simulink model "trail2_SIGNAL_B"  (R2020b)
settings: Solver=FixedStepAuto  StartTime=0.0  StopTime=60  FixedStep=10  RelTol=1e-3
undefined symbols (not defined in the file or in its folder): sigbuilder_block
libraries: simulink x2
settings Model: Creator=99003785  LastModifiedBy=99003785

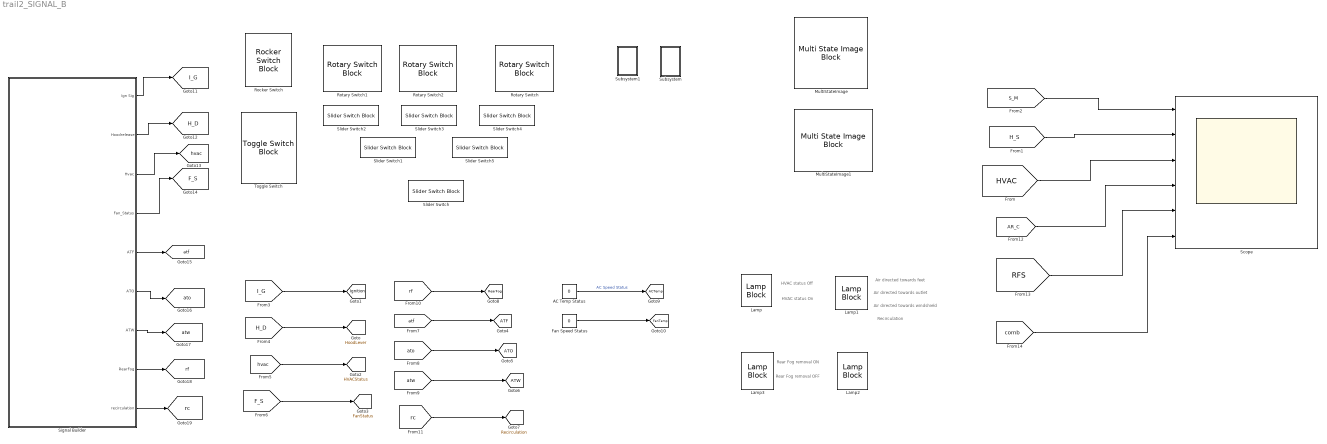
== system trail2_SIGNAL_B ==
  note: Rear Fog removal OFF
  note: Recirculation
  note: Air directed towards feet
  note: Air directed towards outlet
  note: Air directed towards windshield
  note: HVAC status On
  note: Rear Fog removal ON
  note: HVAC status Off
  AC Temp Status : Constant  Value=0
  Fan Speed Status : Constant  Value=0
  Lamp{,1..3} (4 alike) : LampBlock
  MultiStateImage : MultiStateImageBlock
  MultiStateImage1 : MultiStateImageBlock
  Rocker Switch : RockerSwitchBlock
      settings: Values={{'On', 'Off'}, [1 0]}
  Rotary Switch : RotarySwitchBlock
      settings: Values={{'Off', 'Low', 'Medium', 'High'}, [0 1 2 3]}
  Rotary Switch1 : RotarySwitchBlock
      settings: Values={{'Off', 'Low', 'Medium', 'High'}, [0 1 2 3]}
  Rotary Switch2 : RotarySwitchBlock
      settings: Values={{'Off', 'AC', 'Heater', 'Air-Vent'}, [0 1 2 3]}
  Scope : Scope  NumInputPorts=6
  Signal Builder : Subsystem  Tag=STV Subsys  LoadFcn=sigbuilder_block('load');  StartFcn=sigbuilder_block('start');  StopFcn=sigbuilder_block('stop');  ClipboardFcn=sigbuilder_block('clipboard');  mask(Sigbuilder block){tuvar=[0:10]}
      mask help: Simulink:masks:SigbuilderBlock_MD
      mask init:
      | if ~strcmp(get_param(bdroot(gcbh),'SimulationStatus'),'stopped') tuvar = sigbuilder_block('maskInit'); end
      settings: CopyFcn=sigbuilder_block('copy');  DeleteFcn=sigbuilder_block('delete');  ModelCloseFcn=sigbuilder_block('modelClose');  PreSaveFcn=sigbuilder_block('preSave');  PauseFcn=sigbuilder_block('pause');  ContinueFcn=sigbuilder_block('continue');  NameChangeFcn=sigbuilder_block('namechange');  OpenFcn=sigbuilder_block('open',[11.25 5.25 1428 681.75 ]);  CloseFcn=sigbuilder_block('close');
      mask Display: plot(0, 0, 100, 100,[2, 2, 32, 32, 2], [68, 8, 8, 68, 68],[32, 2], [38, 38], [32, 19, 2],[53, 60, 44], [32, 17, 17, 2],[16, 16, 31, 31]);txt = getActiveGroup(gcbh);text(2, 100, txt,'verticalAlignment', 'top');
  Slider Switch{,1..5} (6 alike) : SliderSwitchBlock
      settings: Values={{'Off', 'On'}, [0 1]}
  Subsystem : Subsystem
  Subsystem1 : Subsystem
  Toggle Switch : ToggleSwitchBlock
      settings: Values={{'Off', 'On'}, [0 1]}
  tag scope: ACTemp=global, ATF=global, ATO=global, ATW=global, F_S=global, FanStatus=global, FanTemp=global, HVACStatus=global, H_D=global, HoodLever=global, I_G=global, Ignition=global, RearFog=global, Recirculation=global, atf=global, ato=global, atw=global, hvac=global, rc=global, rf=global
  wires:
  [H_D] -> [HoodLever]
  [I_G] -> [Ignition]
  [hvac] -> [HVACStatus]
  [F_S] -> [FanStatus]
  [atf] -> [ATF]
  [ato] -> [ATO]
  [rf] -> [RearFog]
  [rc] -> [Recirculation]
  [atw] -> [ATW]
  AC Temp Status/1 -> [ACTemp]  "AC Speed Status"
  Fan Speed Status/1 -> [FanTemp]
  [S_M] -> Scope/1
  [H_S] -> Scope/2
  [HVAC] -> Scope/3
  Signal Builder/1(Ign Sig) -> [I_G]
  Signal Builder/2(Hoodrelease) -> [H_D]
  Signal Builder/3(Hvac) -> [hvac]
  Signal Builder/4(Fan_Status) -> [F_S]
  Signal Builder/9(recirculation) -> [rc]
  Signal Builder/8(RearFog) -> [rf]
  Signal Builder/7(ATW) -> [atw]
  Signal Builder/6(ATO) -> [ato]
  Signal Builder/5(ATF) -> [atf]
  [AR_C] -> Scope/4
  [RFS] -> Scope/5
  [comb] -> Scope/6

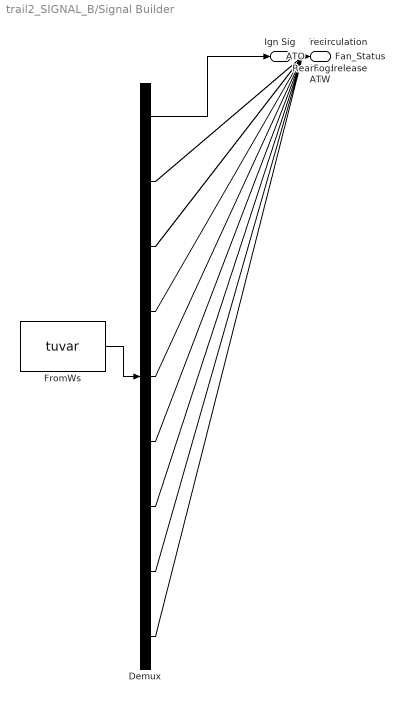
== system trail2_SIGNAL_B/Signal Builder ==
  Demux : Demux  Tag=STV Demux  Outputs=9
      settings: DisplayOption=none
  FromWs : FromWorkspace  Tag=STV FromWs  VariableName=tuvar
      SigBuilderData=|
      | common.afterFinalStr = 'Extrapolate'
      | common.sampleTime = 0
      | dataSet.timeRange = [2 60]
      | dataSet.name = 'Sheet1'
      | sbobj.Groups.Name = 'Sheet1'
      | sbobj.Groups.Signals(1).Name = 'Ign Sig'
      | sbobj.Groups.Signals(1).XData = [2 4 4 8 10 12 14 18 20 22 24 26 28 30 32 34 36 38 40 42 44 45 47 48 50 52 56 58 58 60]
      | sbobj.Groups.Signals(1).YData = [0 0 1 1 1 1 1 1 1 1 1 1 1 1 1 1 1 1 1 1 1 1 1 1 1 1 1 1 0 0]
      | sbobj.Groups.Signals(2).Name = 'Hoodrelease'
      | sbobj.Groups.Signals(2).XData = [2 4 4 8 10 12 14 18 20 22 24 26 28 30 32 34 36 38 40 42 44 45 47 48 50 52 56 58 60]
      | sbobj.Groups.Signals(2).YData = [1 1 0 0 0 0 1 1 1 0 0 0 0 0 0 0 0 0 0 0 0 0 0 0 0 0 0 0 0]
      | sbobj.Groups.Signals(3).Name = 'Hvac'
      | sbobj.Groups.Signals(3).XData = [2 4 4 8 10 10 12 14 18 20 22 24 26 28 30 32 34 36 38 40 42 44 45 47 48 50 52 56 58 58 60]
      | sbobj.Groups.Signals(3).YData = [1 1 0 0 0 1 1 1 1 1 1 1 1 1 1 1 1 1 1 1 1 1 1 1 1 1 1 1 1 0 0]
      | sbobj.Groups.Signals(4).Name = 'Fan_Status'
      | sbobj.Groups.Signals(4).XData = [2 4 8 10 10 12 14 18 20 22 24 26 28 30 32 34 36 38 40 42 44 45 47 48 50 52 56 58 58 60]
      | sbobj.Groups.Signals(4).YData = [0 0 0 0 1 1 1 1 1 1 1 1 1 1 1 1 1 1 1 1 1 1 1 1 1 1 1 1 0 0]
      | sbobj.Groups.Signals(5).Name = 'ATF'
      | sbobj.Groups.Signals(5).XData = [2 4 8 10 12 14 18 20 22 24 26 28 30 32 34 36 38 40 42 44 45 47 48 50 52 56 58 60]
      | sbobj.Groups.Signals(5).YData = [0 0 0 0 0 1 1 1 1 1 0 0 0 0 0 0 0 0 0 0 0 0 0 0 0 0 0 0]
      | sbobj.Groups.Signals(6).Name = 'ATO'
      | sbobj.Groups.Signals(6).XData = [2 4 8 10 10 12 14 18 20 22 24 26 28 30 32 34 36 38 40 42 44 45 47 48 50 52 56 58 60]
      | sbobj.Groups.Signals(6).YData = [0 0 0 0 1 1 1 1 0 0 0 0 0 0 0 0 0 0 0 0 0 0 0 0 0 0 0 0 0]
      | sbobj.Groups.Signals(7).Name = 'ATW'
      | sbobj.Groups.Signals(7).XData = [2 4 8 10 12 14 18 20 22 24 26 28 30 32 34 36 38 40 42 44 45 47 48 50 52 56 58 60]
      | sbobj.Groups.Signals(7).YData = [0 0 0 0 0 1 0 0 0 0 0 1 1 1 1 0 0 0 0 0 0 0 0 0 0 0 0 0]
      | sbobj.Groups.Signals(8).Name = 'RearFog'
      | sbobj.Groups.Signals(8).XData = [2 4 8 10 12 14 18 20 22 24 26 28 30 32 34 36 38 40 42 44 45 47 48 50 52 56 58 60]
      | sbobj.Groups.Signals(8).YData = [0 0 0 0 0 0 0 0 0 0 0 0 0 0 0 1 1 1 1 1 0 0 0 0 0 0 0 0]
      | sbobj.Groups.Signals(9).Name = 'recirculation'
      | sbobj.Groups.Signals(9).XData = [2 4 8 10 12 14 18 20 22 24 26 28 30 32 34 36 38 40 42 44 45 47 48 50 52 56 58 60]
      | sbobj.Groups.Signals(9).YData = [0 0 0 0 0 0 0 0 0 0 0 0 0 0 0 0 0 0 0 0 1 1 1 1 0 0 0 0]
      | sbobj.Groups.TimeRange = [0 20]
  Ign Sig : Outport  Tag=STV Outport
  Hoodrelease : Outport  Tag=STV Outport  Port=2
  Hvac : Outport  Tag=STV Outport  Port=3
  Fan_Status : Outport  Tag=STV Outport  Port=4
  ATF : Outport  Tag=STV Outport  Port=5
  ATO : Outport  Tag=STV Outport  Port=6
  ATW : Outport  Tag=STV Outport  Port=7
  RearFog : Outport  Tag=STV Outport  Port=8
  recirculation : Outport  Tag=STV Outport  Port=9
  wires:
  FromWs/1 -> Demux/1
  Demux/1 -> Ign Sig/1
  Demux/2 -> Hoodrelease/1
  Demux/3 -> Hvac/1
  Demux/4 -> Fan_Status/1
  Demux/5 -> ATF/1
  Demux/6 -> ATO/1
  Demux/7 -> ATW/1
  Demux/8 -> RearFog/1
  Demux/9 -> recirculation/1

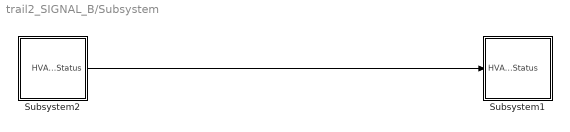
== system trail2_SIGNAL_B/Subsystem ==
  Subsystem1 : Subsystem
  Subsystem2 : Subsystem
  wires:
  Subsystem2/1(HVAC Status) -> Subsystem1/1(HVAC Status)

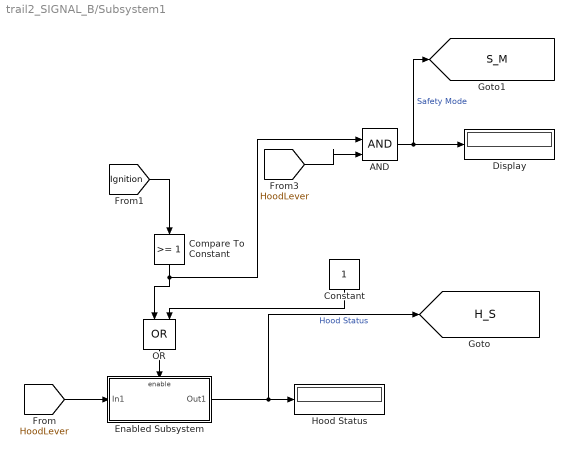
== system trail2_SIGNAL_B/Subsystem1 ==
  AND : Logic  IconShape=distinctive  AllPortsSameDT=off  OutDataTypeStr=boolean
  Compare To Constant : simulink/Logic and Bit Operations/Compare To Constant  relop=>=  const=1  OutDataTypeStr=boolean
  Constant : Constant
  Display : Display
  Enabled Subsystem : Subsystem  TreatAsAtomicUnit=on
  Hood Status : Display
  OR : Logic  Operator=OR  IconShape=distinctive  AllPortsSameDT=off  OutDataTypeStr=boolean
  tag scope: H_S=global, S_M=global
  wires:
  AND/1 -> Display/1, [S_M]  "Safety Mode"
  OR/1 -> Enabled Subsystem/Enable
  Compare To Constant/1 -> AND/1, OR/1
  Constant/1 -> OR/2
  [Ignition] -> Compare To Constant/1
  Enabled Subsystem/1(Out1) -> [H_S], Hood Status/1  "Hood Status"
  [HoodLever] -> Enabled Subsystem/1(In1)
  [HoodLever] -> AND/2

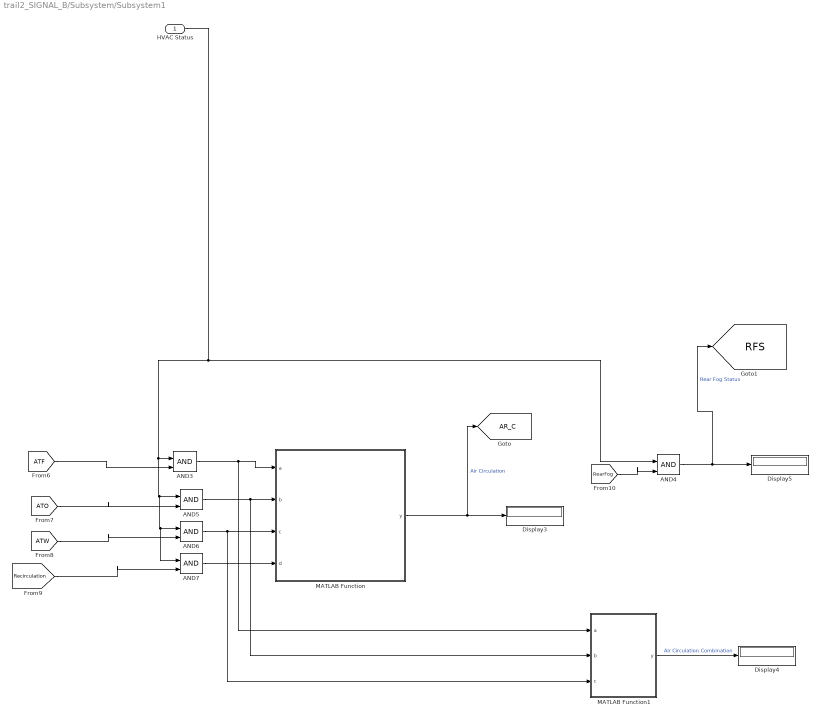
== system trail2_SIGNAL_B/Subsystem/Subsystem1 ==
  HVAC Status : Inport
  AND{3..7} (5 alike) : Logic  IconShape=distinctive  AllPortsSameDT=off  OutDataTypeStr=boolean
  Display3 : Display
  Display4 : Display
  Display5 : Display
  MATLAB Function : MATLAB Function  TreatAsAtomicUnit=on
  MATLAB Function1 : MATLAB Function  TreatAsAtomicUnit=on
  tag scope: AR_C=global, RFS=global
  wires:
  AND3/1 -> MATLAB Function1/1(a), MATLAB Function/1(a)
  AND4/1 -> [RFS], Display5/1  "Rear Fog Status"
  AND6/1 -> MATLAB Function1/3(c), MATLAB Function/3(c)
  AND5/1 -> MATLAB Function1/2(b), MATLAB Function/2(b)
  MATLAB Function1/1(y) -> Display4/1  "Air Circulation Combination"
  AND7/1 -> MATLAB Function/4(d)
  [ATW] -> AND6/2
  [RearFog] -> AND4/2
  [ATO] -> AND5/2
  HVAC Status/1 -> AND7/1, AND6/1, AND5/1, AND3/1, AND4/1
  MATLAB Function/1(y) -> [AR_C], Display3/1  "Air Circulation"
  [Recirculation] -> AND7/2
  [ATF] -> AND3/2

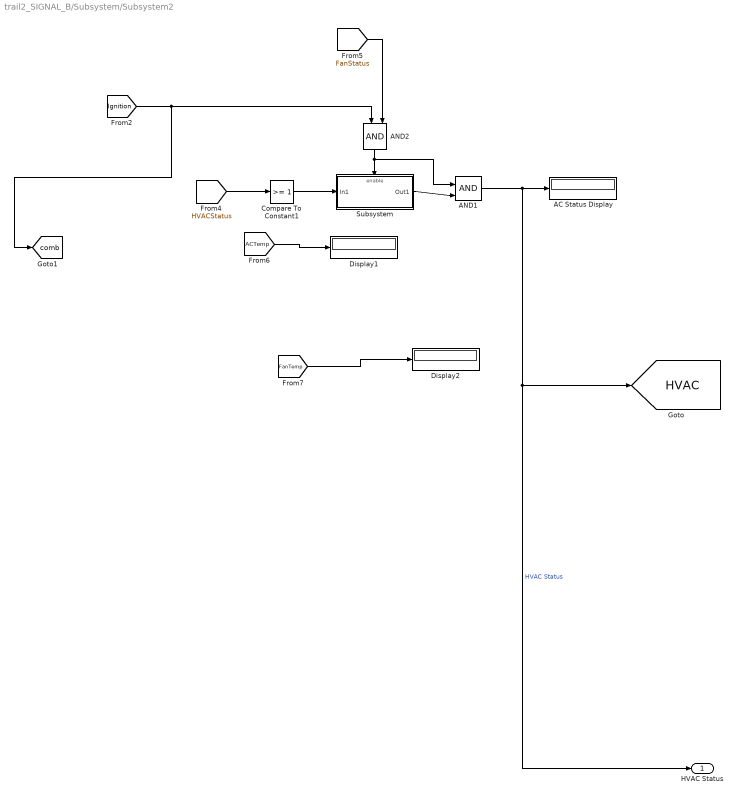
== system trail2_SIGNAL_B/Subsystem/Subsystem2 ==
  AC Status Display : Display
  AND1 : Logic  IconShape=distinctive  AllPortsSameDT=off  OutDataTypeStr=boolean
  AND2 : Logic  IconShape=distinctive  AllPortsSameDT=off  OutDataTypeStr=boolean
  Compare To Constant1 : simulink/Logic and Bit Operations/Compare To Constant  relop=>=  const=1  OutDataTypeStr=boolean
  Display1 : Display
  Display2 : Display
  Subsystem : Subsystem
  HVAC Status : Outport
  tag scope: HVAC=global, comb=global
  wires:
  [FanTemp] -> Display2/1
  [Ignition] -> [comb], AND2/1
  AND1/1 -> [HVAC], HVAC Status/1, AC Status Display/1  "HVAC Status"
  [HVACStatus] -> Compare To Constant1/1
  [ACTemp] -> Display1/1
  [FanStatus] -> AND2/2
  Compare To Constant1/1 -> Subsystem/1(In1)
  AND2/1 -> AND1/1, Subsystem/Enable
  Subsystem/1(Out1) -> AND1/2

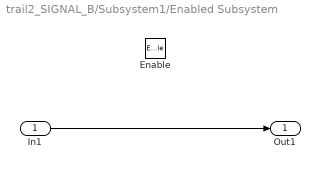
== system trail2_SIGNAL_B/Subsystem1/Enabled Subsystem ==
  In1 : Inport
  Enable : EnablePort
  Out1 : Outport  InitialOutput=0  VectorParamsAs1DForOutWhenUnconnected=off
  wires:
  In1/1 -> Out1/1

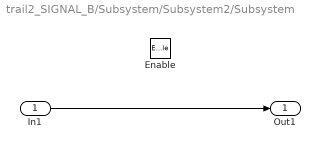
== system trail2_SIGNAL_B/Subsystem/Subsystem2/Subsystem ==
  In1 : Inport
  Enable : EnablePort
  Out1 : Outport
  wires:
  In1/1 -> Out1/1

== matlab function trail2_SIGNAL_B/Subsystem/Subsystem1/MATLAB Function1 ==
  data: a input; b input; c input; y output
function y = fcn(a,b,c)
    if a==1&& b==1 && c==1
        y=1;
    elseif a==1 && b==1 && c==0
        y=2;
    elseif a==1 && b==0 && c==1
        y=3;
    elseif a==0 && b==1 && c==1
        y=4;
    else
        y=0;
    end

end

== matlab function trail2_SIGNAL_B/Subsystem/Subsystem1/MATLAB Function ==
  data: a input; b input; y output; c input; d input
function y = fcn(a, b, c, d)
    if a==1 && b==0 && c==0 && d==0
        y=1;
    elseif a==0 && b==1 &&c==0 && d==0
        y=2;
    elseif a==0 && b==0 &&c==1 && d==0
        y=3;
    elseif a==0 && b==0 &&c==0 && d==1
        y=4;
    else
        y=0;
    end
    

end
